simulink model "lookup_nD_TestGen19"  (R2017b)
settings: Solver=FixedStepDiscrete  StartTime=0.0  StopTime=10.0  RelTol=1e-3
settings Model: Creator=ktrinh  LastModifiedBy=ktrinh
settings DebuggingCC: ParameterOverflowMsg=none

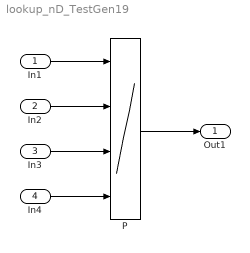
== system lookup_nD_TestGen19 ==
  In1 : Inport  OutMin=0  OutMax=127  OutDataTypeStr=single  PortDimensions=3
  In2 : Inport  Port=2  OutMin=0  OutMax=127  OutDataTypeStr=single
  In3 : Inport  Port=3  OutMin=0  OutMax=127  OutDataTypeStr=single
  In4 : Inport  Port=4  OutMin=0  OutMax=127  OutDataTypeStr=single
  P : Lookup_n-D  NumberOfTableDimensions=4  BreakpointsForDimension1=[55.8726449461824;75.2056601185193]  BreakpointsForDimension2=[12.0790551396318;37.7848385210361;68.3034212566022;69.3247482045485;73.8666780529769]  BreakpointsForDimension3=[35.7911584981003;62.0944319886572;84.2057909296754]  BreakpointsForDimension4=[12.7228046803109;43.5937122702909]  BreakpointsForDimension1DataTypeStr=int8  BreakpointsForDimension2DataTypeStr=int8  BreakpointsForDimension3DataTypeStr=int8  BreakpointsForDimension4DataTypeStr=int8  Table=reshape(repmat([4 5 6 7 8;16 19 20 21 22;10 18 23 24 25],2,2),[2,5,3,2])  InterpMethod=Flat  ExtrapMethod=Clip  UseLastTableValue=on  InternalRulePriority=Speed  OutDataTypeStr=uint32  RndMeth=Simplest  SaturateOnIntegerOverflow=on  InputSameDT=on
  Out1 : Outport
  wires:
  In1/1 -> P/1
  In2/1 -> P/2
  In3/1 -> P/3
  In4/1 -> P/4
  P/1 -> Out1/1
